simulink subsystem "External_Forces"  (R2024a)
settings: Solver=VariableStepAuto  StartTime=0.0  StopTime=10.0  RelTol=1e-3
undefined symbols (not defined in the file): EXT, P0, P1, P10, P2, P3, P4, P5, P6, P7, P8, P9, Sim_param
settings Model: Creator=esben  LastModifiedBy=BP21JL
settings SolverCC: AlgebraicLoopSolver=TrustRegion
settings DebuggingCC: UnconnectedInputMsg=warning  UnconnectedOutputMsg=warning  UnconnectedLineMsg=warning
settings ModelReferenceCC: EnableRefExpFcnMdlSchedulingChecks=on
settings RTWCC: GPUComputeCapability=3.5  DLArmComputeVersion=19.05

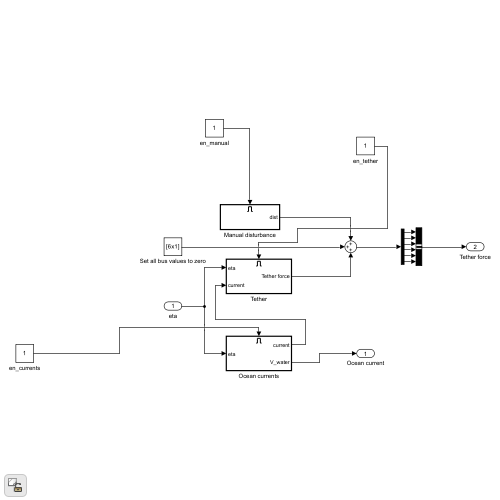
[thumbnail: Simulink's stored preview of the top-level diagram]
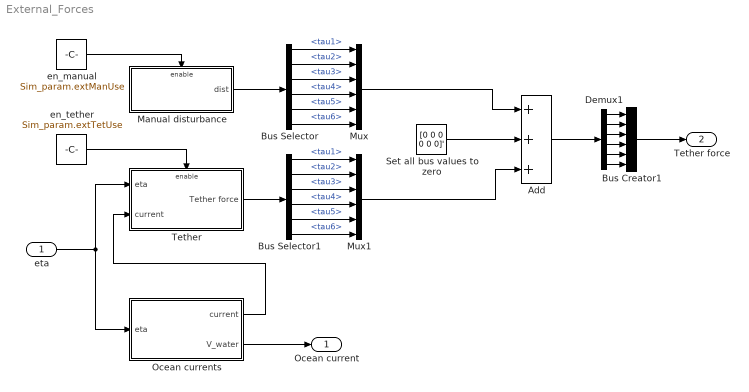
== system External_Forces ==
  eta : Inport
  Add : Sum  Inputs=+++
  Bus Creator1 : BusCreator  Inputs=6  OutDataTypeStr=Bus: tau
  Bus Selector : BusSelector  OutputSignals=tau1,tau2,tau3,tau4,tau5,tau6
  Bus Selector1 : BusSelector  OutputSignals=tau1,tau2,tau3,tau4,tau5,tau6
  Demux1 : Demux  Outputs=6
  Manual disturbance : Subsystem  TreatAsAtomicUnit=on
  Mux : Mux  Inputs=6
  Mux1 : Mux  Inputs=6
  Ocean currents : Subsystem  TreatAsAtomicUnit=on
  Set all bus values to zero : Constant  Value=[0 0 0 0 0 0]'
  Tether : Subsystem  TreatAsAtomicUnit=on
  en_manual : Constant  Value=Sim_param.extManUse
  en_tether : Constant  Value=Sim_param.extTetUse
  Ocean current : Outport
  Tether force : Outport  Port=2
  wires:
  eta/1 -> Tether/1(eta), Ocean currents/1(eta)
  Manual disturbance/1(dist) -> Bus Selector/1
  Demux1/4 -> Bus Creator1/4
  Demux1/2 -> Bus Creator1/2
  Demux1/5 -> Bus Creator1/5
  Demux1/1 -> Bus Creator1/1
  Bus Creator1/1 -> Tether force/1
  Demux1/6 -> Bus Creator1/6
  Demux1/3 -> Bus Creator1/3
  Ocean currents/1(current) -> Tether/2(current)
  Ocean currents/2(V_water) -> Ocean current/1
  en_tether/1 -> Tether/Enable
  en_manual/1 -> Manual disturbance/Enable
  Tether/1(Tether force) -> Bus Selector1/1
  Bus Selector1/1 -> Mux1/1  "<tau1>"
  Bus Selector1/2 -> Mux1/2  "<tau2>"
  Bus Selector1/3 -> Mux1/3  "<tau3>"
  Bus Selector1/4 -> Mux1/4  "<tau4>"
  Bus Selector1/5 -> Mux1/5  "<tau5>"
  Bus Selector1/6 -> Mux1/6  "<tau6>"
  Bus Selector/1 -> Mux/1  "<tau1>"
  Bus Selector/2 -> Mux/2  "<tau2>"
  Bus Selector/3 -> Mux/3  "<tau3>"
  Bus Selector/4 -> Mux/4  "<tau4>"
  Bus Selector/5 -> Mux/5  "<tau5>"
  Bus Selector/6 -> Mux/6  "<tau6>"
  Set all bus values to zero/1 -> Add/2
  Mux/1 -> Add/1
  Mux1/1 -> Add/3
  Add/1 -> Demux1/1

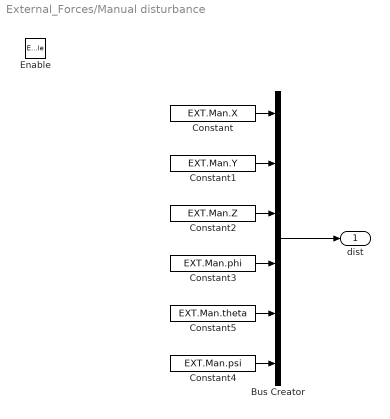
== system External_Forces/Manual disturbance ==
  Enable : EnablePort
  Bus Creator : BusCreator  Inputs=6  OutDataTypeStr=Bus: tau
      settings: InheritFromInputs=off
  Constant : Constant  Value=EXT.Man.X
  Constant1 : Constant  Value=EXT.Man.Y
  Constant2 : Constant  Value=EXT.Man.Z
  Constant3 : Constant  Value=EXT.Man.phi
  Constant4 : Constant  Value=EXT.Man.psi
  Constant5 : Constant  Value=EXT.Man.theta
  dist : Outport  OutDataTypeStr=Bus: tau
  wires:
  Constant1/1 -> Bus Creator/2
  Constant2/1 -> Bus Creator/3
  Constant5/1 -> Bus Creator/5
  Constant/1 -> Bus Creator/1
  Constant4/1 -> Bus Creator/6
  Constant3/1 -> Bus Creator/4
  Bus Creator/1 -> dist/1

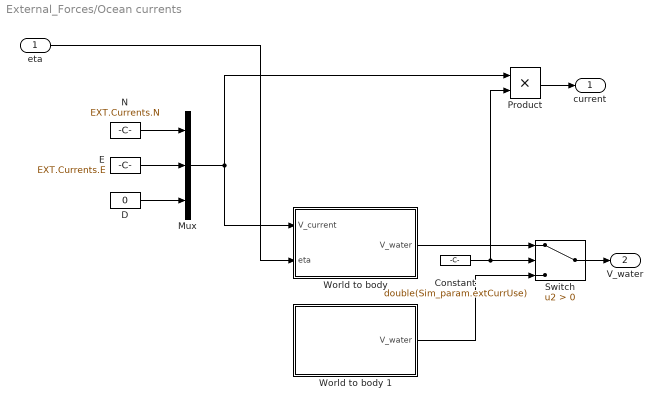
== system External_Forces/Ocean currents ==
  eta : Inport
  Constant : Constant  Value=double(Sim_param.extCurrUse)
  D : Constant  Value=0
  E : Constant  Value=EXT.Currents.E
  Mux : Mux  Inputs=3
  N : Constant  Value=EXT.Currents.N
  Product : Product
  Switch : Switch  Criteria=u2 > Threshold  SaturateOnIntegerOverflow=off  InputSameDT=off
  "World to body " : MATLAB Function  TreatAsAtomicUnit=on
  World to body 1 : MATLAB Function  TreatAsAtomicUnit=on
  current : Outport
  V_water : Outport  Port=2
  wires:
  Switch/1 -> V_water/1
  N/1 -> Mux/1
  eta/1 -> "World to body "/2(eta)
  World to body 1/1(V_water) -> Switch/3
  E/1 -> Mux/2
  "World to body "/1(V_water) -> Switch/1
  Constant/1 -> Switch/2, Product/2
  Product/1 -> current/1
  Mux/1 -> "World to body "/1(V_current), Product/1
  D/1 -> Mux/3

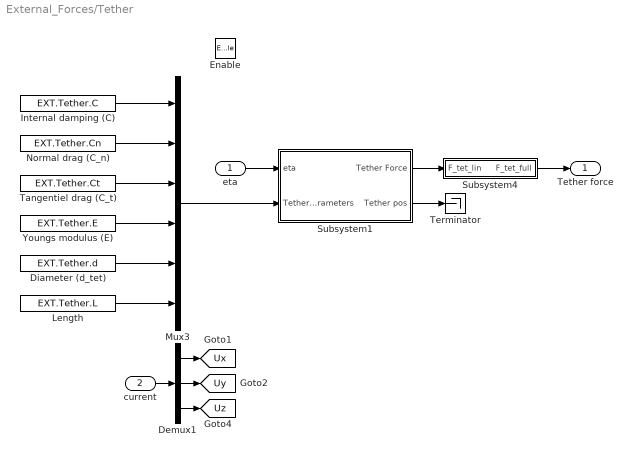
== system External_Forces/Tether ==
  eta : Inport
  current : Inport  Port=2
  Enable : EnablePort
  Demux1 : Demux  Outputs=3
  Diameter (d_tet) : Constant  Value=EXT.Tether.d
  Internal damping (C) : Constant  Value=EXT.Tether.C
  Length : Constant  Value=EXT.Tether.L
  Mux3 : Mux  Inputs=6
  Normal drag (C_n) : Constant  Value=EXT.Tether.Cn
  Subsystem1 : Subsystem
  Subsystem4 : Subsystem
  Tangentiel drag (C_t) : Constant  Value=EXT.Tether.Ct
  Terminator : Terminator
  Youngs modulus (E) : Constant  Value=EXT.Tether.E
  Tether force : Outport  OutDataTypeStr=Bus: tau
  tag scope: Ux=global, Uy=global, Uz=global
  wires:
  Diameter (d_tet)/1 -> Mux3/5
  Length/1 -> Mux3/6
  Demux1/3 -> [Uz]
  Internal damping (C)/1 -> Mux3/1
  Demux1/2 -> [Uy]
  current/1 -> Demux1/1
  Subsystem4/1(F_tet_full) -> Tether force/1
  Subsystem1/2(Tether pos) -> Terminator/1
  Normal drag (C_n)/1 -> Mux3/2
  eta/1 -> Subsystem1/1(eta)
  Mux3/1 -> Subsystem1/2(Tether_Parameters)
  Tangentiel drag (C_t)/1 -> Mux3/3
  Subsystem1/1(Tether Force) -> Subsystem4/1(F_tet_lin)
  Youngs modulus (E)/1 -> Mux3/4
  Demux1/1 -> [Ux]

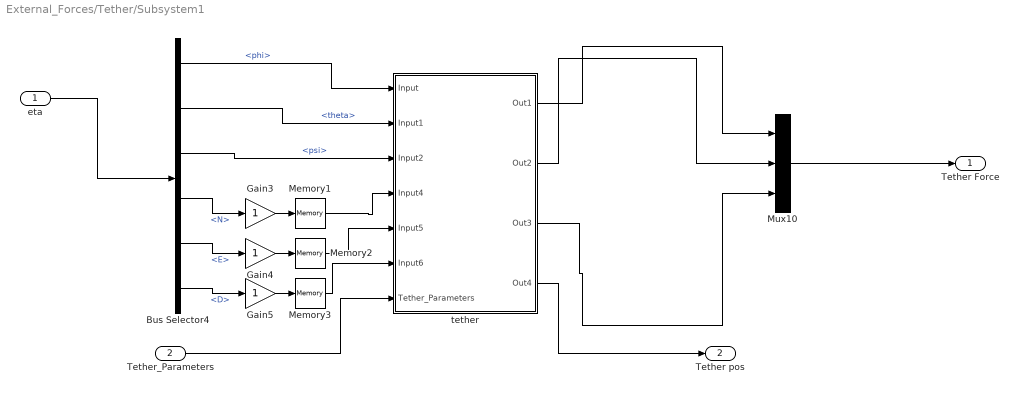
== system External_Forces/Tether/Subsystem1 ==
  eta : Inport
  Tether_Parameters : Inport  Port=2
  Bus Selector4 : BusSelector  OutputSignals=phi,theta,psi,N,E,D
  Gain3 : Gain
  Gain4 : Gain
  Gain5 : Gain
  Memory1 : Memory  InitialCondition=P10(1)
  Memory2 : Memory  InitialCondition=P10(2)
  Memory3 : Memory  InitialCondition=P10(3)
  Mux10 : Mux  Inputs=3
  tether : Subsystem
  Tether Force : Outport
  Tether pos : Outport  Port=2
  wires:
  eta/1 -> Bus Selector4/1
  Bus Selector4/6 -> Gain5/1  "<D>"
  Bus Selector4/5 -> Gain4/1  "<E>"
  Bus Selector4/4 -> Gain3/1  "<N>"
  tether/4(Out4) -> Tether pos/1
  Mux10/1 -> Tether Force/1
  tether/3(Out3) -> Mux10/3
  tether/2(Out2) -> Mux10/2
  tether/1(Out1) -> Mux10/1
  Gain5/1 -> Memory3/1
  Gain4/1 -> Memory2/1
  Gain3/1 -> Memory1/1
  Tether_Parameters/1 -> tether/7(Tether_Parameters)
  Bus Selector4/3 -> tether/3(Input2)  "<psi>"
  Bus Selector4/2 -> tether/2(Input1)  "<theta>"
  Bus Selector4/1 -> tether/1(Input)  "<phi>"
  Memory1/1 -> tether/4(Input4)
  Memory2/1 -> tether/5(Input5)
  Memory3/1 -> tether/6(Input6)

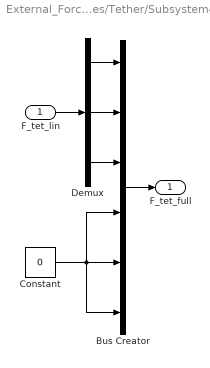
== system External_Forces/Tether/Subsystem4 ==
  F_tet_lin : Inport
  Bus Creator : BusCreator  Inputs=6  OutDataTypeStr=Bus: tau
      settings: InheritFromInputs=off
  Constant : Constant  Value=0
  Demux : Demux  Outputs=3
  F_tet_full : Outport  OutDataTypeStr=Bus: tau
  wires:
  F_tet_lin/1 -> Demux/1
  Demux/3 -> Bus Creator/3
  Demux/2 -> Bus Creator/2
  Demux/1 -> Bus Creator/1
  Bus Creator/1 -> F_tet_full/1
  Constant/1 -> Bus Creator/5, Bus Creator/4, Bus Creator/6

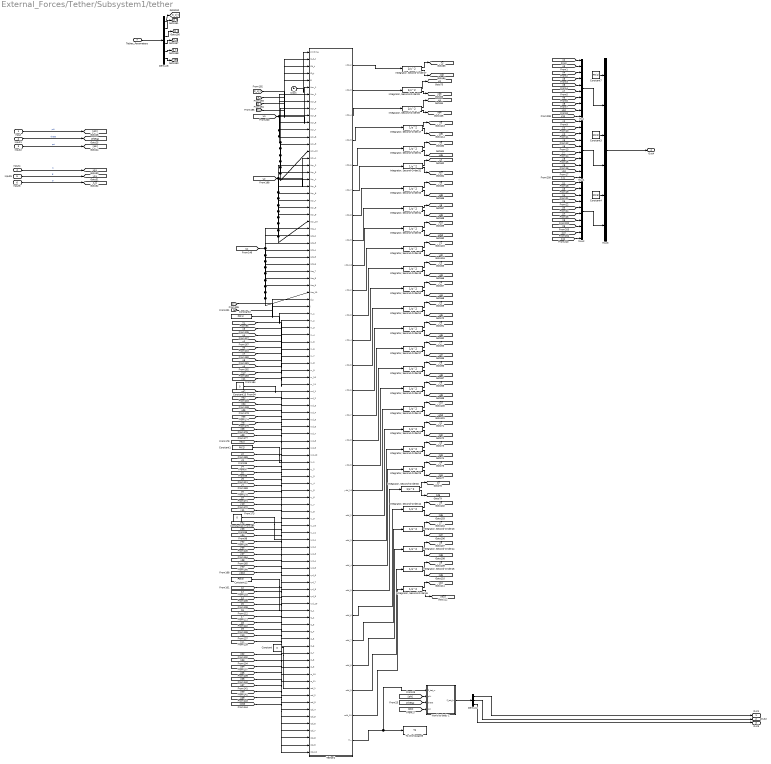
== system External_Forces/Tether/Subsystem1/tether ==
  Input : Inport
  Input1 : Inport  Port=2
  Input2 : Inport  Port=3
  Input4 : Inport  Port=4
  Input5 : Inport  Port=5
  Input6 : Inport  Port=6
  Tether_Parameters : Inport  Port=7
  Clock : Clock
  Constant : Constant  Value=0
  Constant1 : Constant  Value=P0(2)
  Constant10 : Constant  Value=0
  Constant12 : Constant  Value=P0(3)
  Constant13 : Constant  Value=0
  Constant2 : Constant  Value=P0(1)
  Constant3 : Constant  Value=P0(2)
  Constant4 : Constant  Value=P0(3)
  Constant7 : Constant  Value=P0(1)
  Demux4 : Demux  Outputs=3
  Demux6 : Demux  Outputs=6
  "Integrator, Second-Order27" : SecondOrderIntegrator  ICX=P1(1)
  "Integrator, Second-Order28" : SecondOrderIntegrator  ICX=P2(1)
  "Integrator, Second-Order29" : SecondOrderIntegrator  ICX=P3(3)
  "Integrator, Second-Order30" : SecondOrderIntegrator  ICX=P4(3)
  "Integrator, Second-Order31" : SecondOrderIntegrator  ICX=P5(1)
  "Integrator, Second-Order32" : SecondOrderIntegrator  ICX=P6(1)
  "Integrator, Second-Order33" : SecondOrderIntegrator  ICX=P7(1)
  "Integrator, Second-Order34" : SecondOrderIntegrator  ICX=P8(1)  UpperLimitX=100  LowerLimitX=-100  UpperLimitDXDT=10  LowerLimitDXDT=-10
  "Integrator, Second-Order35" : SecondOrderIntegrator  ICX=P9(1)
  "Integrator, Second-Order36" : SecondOrderIntegrator  ICX=P5(2)
  "Integrator, Second-Order37" : SecondOrderIntegrator  ICX=P6(2)
  "Integrator, Second-Order38" : SecondOrderIntegrator  ICX=P7(2)
  "Integrator, Second-Order39" : SecondOrderIntegrator  ICX=P3(1)
  "Integrator, Second-Order40" : SecondOrderIntegrator  ICX=P8(2)
  "Integrator, Second-Order41" : SecondOrderIntegrator  ICX=P9(2)
  "Integrator, Second-Order42" : SecondOrderIntegrator  ICX=P5(3)
  "Integrator, Second-Order43" : SecondOrderIntegrator  ICX=P6(3)
  "Integrator, Second-Order44" : SecondOrderIntegrator  ICX=P7(3)
  "Integrator, Second-Order45" : SecondOrderIntegrator  ICX=P8(3)
  "Integrator, Second-Order46" : SecondOrderIntegrator  ICX=P9(3)
  "Integrator, Second-Order47" : SecondOrderIntegrator  ICX=P4(1)
  "Integrator, Second-Order48" : SecondOrderIntegrator  ICX=P1(2)
  "Integrator, Second-Order49" : SecondOrderIntegrator  ICX=P2(2)
  "Integrator, Second-Order50" : SecondOrderIntegrator  ICX=P3(2)
  "Integrator, Second-Order51" : SecondOrderIntegrator  ICX=P4(2)
  "Integrator, Second-Order52" : SecondOrderIntegrator  ICX=P1(3)
  "Integrator, Second-Order53" : SecondOrderIntegrator  ICX=P2(3)
  Mux : Mux  Inputs=10
  Mux1 : Mux  Inputs=10
  Mux2 : Mux  Inputs=10
  Mux3 : Mux  Inputs=6
  Tether2 : MATLAB Function  TreatAsAtomicUnit=on
  To Workspace3 : ToWorkspace  VariableName=T2  SaveFormat=Timeseries  SampleTime=-1
  World to body 1 : MATLAB Function  TreatAsAtomicUnit=on
  Out1 : Outport
  Out2 : Outport  Port=2
  Out3 : Outport  Port=3
  Out4 : Outport  Port=4
  tag scope: C_d_t=global, Cd_t=global, Ct_t=global, Em_t=global, I_tet=global, d_t=global, x10=global, x11=global, x2=global, x3=global, x4=global, x5=global, x6=global, x7=global, x8=global, x9=global, xd10=global, xd2=global, xd3=global, xd4=global, xd5=global, xd6=global, xd7=global, xd8=global, xd9=global, y10=global, y11=global, y2=global, y3=global, y4=global, y5=global, y6=global, y7=global, y8=global, y9=global, yd10=global, yd2=global, yd3=global, yd4=global, yd5=global, yd6=global, yd7=global, yd8=global, yd9=global, z10=global, z11=global, z2=global, z3=global, z4=global, z5=global, z6=global, z7=global, z8=global, z9=global, zd10=global, zd2=global, zd3=global, zd4=global, zd5=global, zd6=global, zd7=global, zd8=global, zd9=global
  wires:
  Clock/1 -> Tether2/1(simtime)
  Constant4/1 -> Mux3/5
  Constant3/1 -> Mux3/3
  Constant7/1 -> Mux3/1
  Mux3/1 -> Out4/1
  Mux2/1 -> Mux3/6
  Mux1/1 -> Mux3/4
  Mux/1 -> Mux3/2
  [z11] -> Mux2/10
  [y11] -> Mux1/10
  [x11] -> Mux/10
  [z2] -> Mux2/1
  [z6] -> Mux2/5
  [z10] -> Mux2/9
  [z7] -> Mux2/6
  [z8] -> Mux2/7
  [z3] -> Mux2/2
  [z4] -> Mux2/3
  [z5] -> Mux2/4
  [z9] -> Mux2/8
  [y2] -> Mux1/1
  [y6] -> Mux1/5
  [y10] -> Mux1/9
  [y7] -> Mux1/6
  [y8] -> Mux1/7
  [y3] -> Mux1/2
  [y4] -> Mux1/3
  [y5] -> Mux1/4
  [y9] -> Mux1/8
  [x10] -> Mux/9
  [x9] -> Mux/8
  [x8] -> Mux/7
  [x7] -> Mux/6
  [x6] -> Mux/5
  [x5] -> Mux/4
  [x4] -> Mux/3
  [x3] -> Mux/2
  [x2] -> Mux/1
  Constant13/1 -> Tether2/49(rxd_1)
  Constant10/1 -> Tether2/70(ryd_1)
  Constant/1 -> Tether2/91(rzd_1)
  Tether2/4(xdd_5) -> "Integrator, Second-Order47"/1
  Tether2/3(xdd_4) -> "Integrator, Second-Order39"/1
  Tether2/2(xdd_3) -> "Integrator, Second-Order28"/1
  Tether2/1(xdd_2) -> "Integrator, Second-Order27"/1
  Tether2/27(zdd_10) -> "Integrator, Second-Order46"/1
  Tether2/26(zdd_9) -> "Integrator, Second-Order45"/1
  Tether2/25(zdd_8) -> "Integrator, Second-Order44"/1
  Tether2/24(zdd_7) -> "Integrator, Second-Order43"/1
  Tether2/23(zdd_6) -> "Integrator, Second-Order42"/1
  Tether2/22(zdd_5) -> "Integrator, Second-Order30"/1
  Tether2/21(zdd_4) -> "Integrator, Second-Order29"/1
  Tether2/20(zdd_3) -> "Integrator, Second-Order53"/1
  Tether2/19(zdd_2) -> "Integrator, Second-Order52"/1
  Tether2/18(ydd_10) -> "Integrator, Second-Order41"/1
  Tether2/17(ydd_9) -> "Integrator, Second-Order40"/1
  Tether2/16(ydd_8) -> "Integrator, Second-Order38"/1
  Tether2/15(ydd_7) -> "Integrator, Second-Order37"/1
  Tether2/14(ydd_6) -> "Integrator, Second-Order36"/1
  Tether2/13(ydd_5) -> "Integrator, Second-Order51"/1
  Tether2/12(ydd_4) -> "Integrator, Second-Order50"/1
  Tether2/11(ydd_3) -> "Integrator, Second-Order49"/1
  Tether2/10(ydd_2) -> "Integrator, Second-Order48"/1
  Tether2/9(xdd_10) -> "Integrator, Second-Order35"/1
  Tether2/8(xdd_9) -> "Integrator, Second-Order34"/1
  Tether2/7(xdd_8) -> "Integrator, Second-Order33"/1
  Tether2/6(xdd_7) -> "Integrator, Second-Order32"/1
  Tether2/5(xdd_6) -> "Integrator, Second-Order31"/1
  Demux6/1 -> [C_d_t]
  [C_d_t] -> Tether2/2(C_d_t)
  Demux6/4 -> [Em_t]
  Demux6/5 -> [d_t]
  Demux6/2 -> [Cd_t]
  Tether_Parameters/1 -> Demux6/1
  Demux6/3 -> [Ct_t]
  Demux6/6 -> [I_tet]
  [Em_t] -> Tether2/5(E)
  [Ct_t] -> Tether2/4(Ct_t)
  [Cd_t] -> Tether2/3(Cd_t)
  [d_t] -> Tether2/36(d_t)
  [Uy] -> Tether2/16(Ucy_1), Tether2/17(Ucy_2), Tether2/18(Ucy_3), Tether2/19(Ucy_4), Tether2/20(Ucy_5), Tether2/21(Ucy_6), Tether2/22(Ucy_7), Tether2/23(Ucy_8), Tether2/24(Ucy_9), Tether2/25(Ucy_10)
  Demux4/2 -> Out2/1
  Demux4/3 -> Out3/1
  Demux4/1 -> Out1/1
  Tether2/28(Tix) -> To Workspace3/1, World to body 1/1(F_tet_w)
  [phi] -> World to body 1/2(phi)
  [theta] -> World to body 1/3(theta)
  World to body 1/1(F_tet_b) -> Demux4/1
  [psi] -> World to body 1/4(psi)
  [I_tet] -> Tether2/37(l)
  [Ux] -> Tether2/6(Ucx_1), Tether2/7(Ucx_2), Tether2/8(Ucx_3), Tether2/9(Ucx_4), Tether2/10(Ucx_5), Tether2/11(Ucx_6), Tether2/12(Ucx_7), Tether2/13(Ucx_8), Tether2/14(Ucx_9), Tether2/15(Ucx_10)
  [x9] -> Tether2/46(rx_9)
  "Integrator, Second-Order42"/1 -> [z6]
  [y3] -> Tether2/61(ry_3)
  "Integrator, Second-Order53"/2 -> [zd3]
  "Integrator, Second-Order43"/2 -> [zd7]
  [xd2] -> Tether2/50(rxd_2)
  "Integrator, Second-Order38"/2 -> [yd8]
  "Integrator, Second-Order39"/2 -> [xd4]
  "Integrator, Second-Order33"/1 -> [x8]
  [x11] -> Tether2/48(rx_11)
  [Uz] -> Tether2/26(Ucz_1), Tether2/27(Ucz_2), Tether2/28(Ucz_3), Tether2/29(Ucz_4), Tether2/30(Ucz_5), Tether2/31(Ucz_6), Tether2/32(Ucz_7), Tether2/33(Ucz_8), Tether2/34(Ucz_9), Tether2/35(Ucz_10)
  [x2] -> Tether2/39(rx_2)
  [x10] -> Tether2/47(rx_10)
  "Integrator, Second-Order42"/2 -> [zd6]
  [z10] -> Tether2/89(rz_10)
  [y8] -> Tether2/66(ry_8)
  [yd9] -> Tether2/78(ryd_9)
  [xd7] -> Tether2/55(rxd_7)
  [y11] -> Tether2/69(ry_11)
  "Integrator, Second-Order27"/2 -> [xd2]
  "Integrator, Second-Order49"/2 -> [yd3]
  [y2] -> Tether2/60(ry_2)
  "Integrator, Second-Order30"/2 -> [zd5]
  [xd3] -> Tether2/51(rxd_3)
  "Integrator, Second-Order35"/1 -> [x10]
  [zd2] -> Tether2/92(rzd_2)
  [yd6] -> Tether2/75(ryd_6)
  [y7] -> Tether2/65(ry_7)
  [x5] -> Tether2/42(rx_5)
  [xd10] -> Tether2/58(rxd_10)
  [x8] -> Tether2/45(rx_8)
  [zd8] -> Tether2/98(rzd_8)
  [x6] -> Tether2/43(rx_6)
  [yd4] -> Tether2/73(ryd_4)
  "Integrator, Second-Order34"/2 -> [xd9]
  [xd6] -> Tether2/54(rxd_6)
  [z2] -> Tether2/81(rz_2)
  [z7] -> Tether2/86(rz_7)
  "Integrator, Second-Order39"/1 -> [x4]
  [z5] -> Tether2/84(rz_5)
  "Integrator, Second-Order28"/1 -> [x3]
  "Integrator, Second-Order44"/1 -> [z8]
  "Integrator, Second-Order34"/1 -> [x9]
  Constant2/1 -> Tether2/38(rx_1)
  "Integrator, Second-Order51"/1 -> [y5]
  "Integrator, Second-Order43"/1 -> [z7]
  "Integrator, Second-Order40"/2 -> [yd9]
  [z6] -> Tether2/85(rz_6)
  "Integrator, Second-Order37"/1 -> [y7]
  [xd8] -> Tether2/56(rxd_8)
  "Integrator, Second-Order45"/1 -> [z9]
  [x4] -> Tether2/41(rx_4)
  "Integrator, Second-Order32"/2 -> [xd7]
  "Integrator, Second-Order49"/1 -> [y3]
  "Integrator, Second-Order47"/1 -> [x5]
  "Integrator, Second-Order36"/2 -> [yd6]
  "Integrator, Second-Order51"/2 -> [yd5]
  [yd2] -> Tether2/71(ryd_2)
  "Integrator, Second-Order48"/2 -> [yd2]
  "Integrator, Second-Order27"/1 -> [x2]
  "Integrator, Second-Order40"/1 -> [y9]
  "Integrator, Second-Order44"/2 -> [zd8]
  [yd5] -> Tether2/74(ryd_5)
  [x3] -> Tether2/40(rx_3)
  [zd9] -> Tether2/99(rzd_9)
  [x7] -> Tether2/44(rx_7)
  "Integrator, Second-Order37"/2 -> [yd7]
  [xd4] -> Tether2/52(rxd_4)
  [z3] -> Tether2/82(rz_3)
  "Integrator, Second-Order31"/1 -> [x6]
  [y4] -> Tether2/62(ry_4)
  "Integrator, Second-Order47"/2 -> [xd5]
  [z11] -> Tether2/90(rz_11)
  [zd4] -> Tether2/94(rzd_4)
  "Integrator, Second-Order45"/2 -> [zd9]
  "Integrator, Second-Order48"/1 -> [y2]
  [y10] -> Tether2/68(ry_10)
  [z4] -> Tether2/83(rz_4)
  [yd10] -> Tether2/79(ryd_10)
  "Integrator, Second-Order46"/2 -> [zd10]
  [y9] -> Tether2/67(ry_9)
  Constant1/1 -> Tether2/59(ry_1)
  "Integrator, Second-Order30"/1 -> [z5]
  "Integrator, Second-Order41"/1 -> [y10]
  [yd8] -> Tether2/77(ryd_8)
  "Integrator, Second-Order33"/2 -> [xd8]
  "Integrator, Second-Order31"/2 -> [xd6]
  "Integrator, Second-Order38"/1 -> [y8]
  [z9] -> Tether2/88(rz_9)
  "Integrator, Second-Order41"/2 -> [yd10]
  [yd3] -> Tether2/72(ryd_3)
  [zd6] -> Tether2/96(rzd_6)
  [xd9] -> Tether2/57(rxd_9)
  [zd10] -> Tether2/100(rzd_10)
  [zd5] -> Tether2/95(rzd_5)
  "Integrator, Second-Order53"/1 -> [z3]
  "Integrator, Second-Order50"/2 -> [yd4]
  [xd5] -> Tether2/53(rxd_5)
  [y6] -> Tether2/64(ry_6)
  "Integrator, Second-Order50"/1 -> [y4]
  [z8] -> Tether2/87(rz_8)
  "Integrator, Second-Order52"/2 -> [zd2]
  [y5] -> Tether2/63(ry_5)
  "Integrator, Second-Order35"/2 -> [xd10]
  "Integrator, Second-Order29"/1 -> [z4]
  "Integrator, Second-Order29"/2 -> [zd4]
  Constant12/1 -> Tether2/80(rz_1)
  [zd3] -> Tether2/93(rzd_3)
  [yd7] -> Tether2/76(ryd_7)
  "Integrator, Second-Order32"/1 -> [x7]
  "Integrator, Second-Order36"/1 -> [y6]
  "Integrator, Second-Order28"/2 -> [xd3]
  [zd7] -> Tether2/97(rzd_7)
  "Integrator, Second-Order52"/1 -> [z2]
  "Integrator, Second-Order46"/1 -> [z10]
  Input6/1 -> [z11]  "D"
  Input5/1 -> [y11]  "E"
  Input4/1 -> [x11]  "N"
  Input2/1 -> [psi]  "psi"
  Input1/1 -> [theta]  "theta"
  Input/1 -> [phi]  "phi"

== matlab function External_Forces/Tether/Subsystem1/tether/Tether2 ==
  data: simtime input; C_d_t input; xdd_2 output; Cd_t input; Ct_t input; E input; Ucx_1 input; Ucx_2 input; Ucx_3 input; Ucx_4 input; Ucx_5 input; Ucx_6 input; Ucx_7 input; Ucx_8 input; Ucx_9 input; Ucx_10 input; Ucy_1 input; Ucy_2 input; Ucy_3 input; Ucy_4 input; Ucy_5 input; Ucy_6 input; Ucy_7 input; Ucy_8 input; Ucy_9 input; Ucy_10 input; Ucz_1 input; Ucz_2 input; Ucz_3 input; Ucz_4 input; Ucz_5 input; Ucz_6 input; Ucz_7 input; Ucz_8 input; Ucz_9 input; Ucz_10 input; d_t input; l input; rx_1 input; rx_2 input; rx_3 input; rx_4 input; rx_5 input; rx_6 input; rx_7 input; rx_8 input; rx_9 input; rx_10 input; rx_11 input; rxd_1 input; rxd_2 input; rxd_3 input; rxd_4 input; rxd_5 input; rxd_6 input; rxd_7 input; rxd_8 input; rxd_9 input; rxd_10 input; ry_1 input; ry_2 input; ry_3 input; ry_4 input; ry_5 input; ry_6 input; ry_7 input; ry_8 input; ry_9 input; ry_10 input; ry_11 input; ryd_1 input; ryd_2 input; ryd_3 input; ryd_4 input; ryd_5 input; ryd_6 input; ryd_7 input; ryd_8 input; ryd_9 input; ryd_10 input; rz_1 input; rz_2 input; rz_3 input; rz_4 input; rz_5 input; rz_6 input; rz_7 input; rz_8 input; rz_9 input; rz_10 input; rz_11 input; rzd_1 input; rzd_2 input; rzd_3 input; rzd_4 input; rzd_5 input; rzd_6 input; rzd_7 input; rzd_8 input; rzd_9 input; rzd_10 input; xdd_3 output; xdd_4 output; xdd_5 output; xdd_6 output; xdd_7 output; xdd_8 output; xdd_9 output; xdd_10 output; ydd_2 output; ydd_3 output; ydd_4 output; ydd_5 output; ydd_6 output; ydd_7 output; ydd_8 output; ydd_9 output; ydd_10 output; zdd_2 output; zdd_3 output; zdd_4 output; zdd_5 output; zdd_6 output; zdd_7 output; zdd_8 output; zdd_9 output; zdd_10 output; Tix output
function [xdd_2,xdd_3,xdd_4,xdd_5,xdd_6,xdd_7,xdd_8,xdd_9,xdd_10,ydd_2,ydd_3,ydd_4,ydd_5,ydd_6,ydd_7,ydd_8,ydd_9,ydd_10,zdd_2,zdd_3,zdd_4,zdd_5,zdd_6,zdd_7,zdd_8,zdd_9,zdd_10,Tix] = Tether(simtime,C_d_t,Cd_t,Ct_t,E,Ucx_1,Ucx_2,Ucx_3,Ucx_4,Ucx_5,Ucx_6,Ucx_7,Ucx_8,Ucx_9,Ucx_10,Ucy_1,Ucy_2,Ucy_3,Ucy_4,Ucy_5,Ucy_6,Ucy_7,Ucy_8,Ucy_9,Ucy_10,Ucz_1,Ucz_2,Ucz_3,Ucz_4,Ucz_5,Ucz_6,Ucz_7,Ucz_8,Ucz_9,Ucz_10,d_t,l,rx_1,rx_2,rx_3,rx_4,rx_5,rx_6,rx_7,rx_8,rx_9,rx_10,rx_11,rxd_1,rxd_2,rxd_3,rxd_4,rxd_5,rxd_6,rxd_7,rxd_8,rxd_9,rxd_10,ry_1,ry_2,ry_3,ry_4,ry_5,ry_6,ry_7,ry_8,ry_9,ry_10,ry_11,ryd_1,ryd_2,ryd_3,ryd_4,ryd_5,ryd_6,ryd_7,ryd_8,ryd_9,ryd_10,rz_1,rz_2,rz_3,rz_4,rz_5,rz_6,rz_7,rz_8,rz_9,rz_10,rz_11,rzd_1,rzd_2,rzd_3,rzd_4,rzd_5,rzd_6,rzd_7,rzd_8,rzd_9,rzd_10)
%#codegen

%    This function was generated by the Symbolic Math Toolbox version 8.6.
%    17-Mar-2022 13:31:39
%if simtime > 0.5

t2 = d_t.^2;
t3 = -Ucx_2;
t4 = -Ucx_3;
t5 = -Ucx_4;
t6 = -Ucx_5;
t7 = -Ucx_6;
t8 = -Ucx_7;
t9 = -Ucx_8;
t10 = -Ucx_9;
t11 = -Ucx_10;
t12 = -Ucy_2;
t13 = -Ucy_3;
t14 = -Ucy_4;
t15 = -Ucy_5;
t16 = -Ucy_6;
t17 = -Ucy_7;
t18 = -Ucy_8;
t19 = -Ucy_9;
t20 = -Ucy_10;
t21 = -Ucz_2;
t22 = -Ucz_3;
t23 = -Ucz_4;
t24 = -Ucz_5;
t25 = -Ucz_6;
t26 = -Ucz_7;
t27 = -Ucz_8;
t28 = -Ucz_9;
t29 = -Ucz_10;
t30 = 1.0./l;
t31 = -rx_2;
t32 = -rx_3;
t33 = -rx_4;
t34 = -rx_5;
t35 = -rx_6;
t36 = -rx_7;
t37 = -rx_8;
t38 = -rx_9;
t39 = -rx_10;
t40 = -rx_11;
t41 = -rxd_2;
t42 = -rxd_3;
t43 = -rxd_4;
t44 = -rxd_5;
t45 = -rxd_6;
t46 = -rxd_7;
t47 = -rxd_8;
t48 = -rxd_9;
t49 = -rxd_10;
t50 = -ry_2;
t51 = -ry_3;
t52 = -ry_4;
t53 = -ry_5;
t54 = -ry_6;
t55 = -ry_7;
t56 = -ry_8;
t57 = -ry_9;
t58 = -ry_10;
t59 = -ry_11;
t60 = -ryd_2;
t61 = -ryd_3;
t62 = -ryd_4;
t63 = -ryd_5;
t64 = -ryd_6;
t65 = -ryd_7;
t66 = -ryd_8;
t67 = -ryd_9;
t68 = -ryd_10;
t69 = -rz_2;
t70 = -rz_3;
t71 = -rz_4;
t72 = -rz_5;
t73 = -rz_6;
t74 = -rz_7;
t75 = -rz_8;
t76 = -rz_9;
t77 = -rz_10;
t78 = -rz_11;
t79 = -rzd_2;
t80 = -rzd_3;
t81 = -rzd_4;
t82 = -rzd_5;
t83 = -rzd_6;
t84 = -rzd_7;
t85 = -rzd_8;
t86 = -rzd_9;
t87 = -rzd_10;
t260 = l.*4.3e-3;
t88 = Ucx_2+t41;
t89 = Ucx_3+t42;
t90 = Ucx_4+t43;
t91 = Ucx_5+t44;
t92 = Ucx_6+t45;
t93 = Ucx_7+t46;
t94 = Ucx_8+t47;
t95 = Ucx_9+t48;
t96 = Ucx_10+t49;
t97 = Ucy_2+t60;
t98 = Ucy_3+t61;
t99 = Ucy_4+t62;
t100 = Ucy_5+t63;
t101 = Ucy_6+t64;
t102 = Ucy_7+t65;
t103 = Ucy_8+t66;
t104 = Ucy_9+t67;
t105 = Ucy_10+t68;
t106 = Ucz_2+t79;
t107 = Ucz_3+t80;
t108 = Ucz_4+t81;
t109 = Ucz_5+t82;
t110 = Ucz_6+t83;
t111 = Ucz_7+t84;
t112 = Ucz_8+t85;
t113 = Ucz_9+t86;
t114 = Ucz_10+t87;
t115 = rx_1+t31;
t116 = rx_2+t32;
t117 = rx_3+t33;
t118 = rx_4+t34;
t119 = rx_5+t35;
t120 = rx_6+t36;
t121 = rx_7+t37;
t122 = rx_8+t38;
t123 = rx_9+t39;
t124 = rx_10+t40;
t125 = rxd_1+t41;
t126 = rxd_2+t42;
t127 = rxd_3+t43;
t128 = rxd_4+t44;
t129 = rxd_5+t45;
t130 = rxd_6+t46;
t131 = rxd_7+t47;
t132 = rxd_8+t48;
t133 = rxd_9+t49;
t134 = ry_1+t50;
t135 = ry_2+t51;
t136 = ry_3+t52;
t137 = ry_4+t53;
t138 = ry_5+t54;
t139 = ry_6+t55;
t140 = ry_7+t56;
t141 = ry_8+t57;
t142 = ry_9+t58;
t143 = ry_10+t59;
t144 = ryd_1+t60;
t145 = ryd_2+t61;
t146 = ryd_3+t62;
t147 = ryd_4+t63;
t148 = ryd_5+t64;
t149 = ryd_6+t65;
t150 = ryd_7+t66;
t151 = ryd_8+t67;
t152 = ryd_9+t68;
t153 = rz_1+t69;
t154 = rz_2+t70;
t155 = rz_3+t71;
t156 = rz_4+t72;
t157 = rz_5+t73;
t158 = rz_6+t74;
t159 = rz_7+t75;
t160 = rz_8+t76;
t161 = rz_9+t77;
t162 = rz_10+t78;
t163 = rzd_1+t79;
t164 = rzd_2+t80;
t165 = rzd_3+t81;
t166 = rzd_4+t82;
t167 = rzd_5+t83;
t168 = rzd_6+t84;
t169 = rzd_7+t85;
t170 = rzd_8+t86;
t171 = rzd_9+t87;
t229 = l.*t2.*pi.*2.5e+1;
t172 = abs(t115);
t173 = abs(t116);
t174 = abs(t117);
t175 = abs(t118);
t176 = abs(t119);
t177 = abs(t120);
t178 = abs(t121);
t179 = abs(t122);
t180 = abs(t123);
t181 = abs(t124);
t182 = abs(t134);
t183 = abs(t135);
t184 = abs(t136);
t185 = abs(t137);
t186 = abs(t138);
t187 = abs(t139);
t188 = abs(t140);
t189 = abs(t141);
t190 = abs(t142);
t191 = abs(t143);
t192 = abs(t153);
t193 = abs(t154);
t194 = abs(t155);
t195 = abs(t156);
t196 = abs(t157);
t197 = abs(t158);
t198 = abs(t159);
t199 = abs(t160);
t200 = abs(t161);
t201 = abs(t162);
t202 = t115.^2;
t203 = t116.^2;
t204 = t117.^2;
t205 = t118.^2;
t206 = t119.^2;
t207 = t120.^2;
t208 = t121.^2;
t209 = t122.^2;
t210 = t123.^2;
t211 = t134.^2;
t212 = t135.^2;
t213 = t136.^2;
t214 = t137.^2;
t215 = t138.^2;
t216 = t139.^2;
t217 = t140.^2;
t218 = t141.^2;
t219 = t142.^2;
t220 = t153.^2;
t221 = t154.^2;
t222 = t155.^2;
t223 = t156.^2;
t224 = t157.^2;
t225 = t158.^2;
t226 = t159.^2;
t227 = t160.^2;
t228 = t161.^2;
t261 = rxd_1.*t30.*t115.*1.0e+1;
t262 = ryd_1.*t30.*t134.*1.0e+1;
t263 = rzd_1.*t30.*t153.*1.0e+1;
t264 = t229+t260;
t265 = t30.*t116.*t125.*1.0e+1;
t266 = t30.*t117.*t126.*1.0e+1;
t267 = t30.*t118.*t127.*1.0e+1;
t268 = t30.*t119.*t128.*1.0e+1;
t269 = t30.*t120.*t129.*1.0e+1;
t270 = t30.*t121.*t130.*1.0e+1;
t271 = t30.*t122.*t131.*1.0e+1;
t272 = t30.*t123.*t132.*1.0e+1;
t273 = t30.*t124.*t133.*1.0e+1;
t274 = t30.*t135.*t144.*1.0e+1;
t275 = t30.*t136.*t145.*1.0e+1;
t276 = t30.*t137.*t146.*1.0e+1;
t277 = t30.*t138.*t147.*1.0e+1;
t278 = t30.*t139.*t148.*1.0e+1;
t279 = t30.*t140.*t149.*1.0e+1;
t280 = t30.*t141.*t150.*1.0e+1;
t281 = t30.*t142.*t151.*1.0e+1;
t282 = t30.*t143.*t152.*1.0e+1;
t283 = t30.*t154.*t163.*1.0e+1;
t284 = t30.*t155.*t164.*1.0e+1;
t285 = t30.*t156.*t165.*1.0e+1;
t286 = t30.*t157.*t166.*1.0e+1;
t287 = t30.*t158.*t167.*1.0e+1;
t288 = t30.*t159.*t168.*1.0e+1;
t289 = t30.*t160.*t169.*1.0e+1;
t290 = t30.*t161.*t170.*1.0e+1;
t291 = t30.*t162.*t171.*1.0e+1;
t230 = t172.^2;
t231 = t173.^2;
t232 = t174.^2;
t233 = t175.^2;
t234 = t176.^2;
t235 = t177.^2;
t236 = t178.^2;
t237 = t179.^2;
t238 = t180.^2;
t239 = t181.^2;
t240 = t182.^2;
t241 = t183.^2;
t242 = t184.^2;
t243 = t185.^2;
t244 = t186.^2;
t245 = t187.^2;
t246 = t188.^2;
t247 = t189.^2;
t248 = t190.^2;
t249 = t191.^2;
t250 = t192.^2;
t251 = t193.^2;
t252 = t194.^2;
t253 = t195.^2;
t254 = t196.^2;
t255 = t197.^2;
t256 = t198.^2;
t257 = t199.^2;
t258 = t200.^2;
t259 = t201.^2;
t292 = 1.0./t264;
t363 = t261+t262+t263;
t415 = t265+t274+t283;
t416 = t266+t275+t284;
t417 = t267+t276+t285;
t418 = t268+t277+t286;
t419 = t269+t278+t287;
t420 = t270+t279+t288;
t421 = t271+t280+t289;
t422 = t272+t281+t290;
t423 = t273+t282+t291;
t293 = t230+t240+t250;
t294 = t231+t241+t251;
t295 = t232+t242+t252;
t296 = t233+t243+t253;
t297 = t234+t244+t254;
t298 = t235+t245+t255;
t299 = t236+t246+t256;
t300 = t237+t247+t257;
t301 = t238+t248+t258;
t302 = t239+t249+t259;
t303 = 1.0./t293;
t304 = 1.0./t294;
t306 = 1.0./t295;
t308 = 1.0./t296;
t310 = 1.0./t297;
t312 = 1.0./t298;
t314 = 1.0./t299;
t316 = 1.0./t300;
t318 = 1.0./t301;
t320 = 1.0./t302.^2;
t321 = sqrt(t294);
t322 = sqrt(t295);
t323 = sqrt(t296);
t324 = sqrt(t297);
t325 = sqrt(t298);
t326 = sqrt(t299);
t327 = sqrt(t300);
t328 = sqrt(t301);
t329 = sqrt(t302);
t330 = 1.0./sqrt(t293);
t305 = t304.^2;
t307 = t306.^2;
t309 = t308.^2;
t311 = t310.^2;
t313 = t312.^2;
t315 = t314.^2;
t317 = t316.^2;
t319 = t318.^2;
t331 = 1.0./t321;
t332 = 1.0./t322;
t333 = 1.0./t323;
t334 = 1.0./t324;
t335 = 1.0./t325;
t336 = 1.0./t326;
t337 = 1.0./t327;
t338 = 1.0./t328;
t339 = 1.0./t329;
t340 = (l.*t330)./1.0e+1;
t350 = Ucx_1.*t202.*t303;
t351 = Ucy_1.*t211.*t303;
t352 = Ucz_1.*t220.*t303;
t364 = t88.*t203.*t304;
t365 = t89.*t204.*t306;
t366 = t90.*t205.*t308;
t367 = t91.*t206.*t310;
t368 = t92.*t207.*t312;
t369 = t93.*t208.*t314;
t370 = t94.*t209.*t316;
t371 = t95.*t210.*t318;
t372 = t97.*t212.*t304;
t373 = t98.*t213.*t306;
t374 = t99.*t214.*t308;
t375 = t100.*t215.*t310;
t376 = t101.*t216.*t312;
t377 = t102.*t217.*t314;
t378 = t103.*t218.*t316;
t379 = t104.*t219.*t318;
t380 = t106.*t221.*t304;
t381 = t107.*t222.*t306;
t382 = t108.*t223.*t308;
t383 = t109.*t224.*t310;
t384 = t110.*t225.*t312;
t385 = t111.*t226.*t314;
t386 = t112.*t227.*t316;
t387 = t113.*t228.*t318;
t341 = (l.*t331)./1.0e+1;
t342 = (l.*t332)./1.0e+1;
t343 = (l.*t333)./1.0e+1;
t344 = (l.*t334)./1.0e+1;
t345 = (l.*t335)./1.0e+1;
t346 = (l.*t336)./1.0e+1;
t347 = (l.*t337)./1.0e+1;
t348 = (l.*t338)./1.0e+1;
t349 = (l.*t339)./1.0e+1;
t353 = t340-1.0;
t388 = rxd_2+t3+t350;
t389 = ryd_2+t12+t351;
t390 = rzd_2+t21+t352;
t391 = rxd_3+t4+t364;
t392 = rxd_4+t5+t365;
t393 = rxd_5+t6+t366;
t394 = rxd_6+t7+t367;
t395 = rxd_7+t8+t368;
t396 = rxd_8+t9+t369;
t397 = rxd_9+t10+t370;
t398 = rxd_10+t11+t371;
t399 = ryd_3+t13+t372;
t400 = ryd_4+t14+t373;
t401 = ryd_5+t15+t374;
t402 = ryd_6+t16+t375;
t403 = ryd_7+t17+t376;
t404 = ryd_8+t18+t377;
t405 = ryd_9+t19+t378;
t406 = ryd_10+t20+t379;
t407 = rzd_3+t22+t380;
t408 = rzd_4+t23+t381;
t409 = rzd_5+t24+t382;
t410 = rzd_6+t25+t383;
t411 = rzd_7+t26+t384;
t412 = rzd_8+t27+t385;
t413 = rzd_9+t28+t386;
t414 = rzd_10+t29+t387;
t451 = C_d_t.*t116.*t331.*t415;
t452 = C_d_t.*t117.*t332.*t416;
t453 = C_d_t.*t118.*t333.*t417;
t454 = C_d_t.*t119.*t334.*t418;
t455 = C_d_t.*t120.*t335.*t419;
t456 = C_d_t.*t121.*t336.*t420;
t457 = C_d_t.*t122.*t337.*t421;
t458 = C_d_t.*t123.*t338.*t422;
t459 = C_d_t.*t135.*t331.*t415;
t460 = C_d_t.*t136.*t332.*t416;
t461 = C_d_t.*t137.*t333.*t417;
t462 = C_d_t.*t138.*t334.*t418;
t463 = C_d_t.*t139.*t335.*t419;
t464 = C_d_t.*t140.*t336.*t420;
t465 = C_d_t.*t141.*t337.*t421;
t466 = C_d_t.*t142.*t338.*t422;
t467 = C_d_t.*t154.*t331.*t415;
t468 = C_d_t.*t155.*t332.*t416;
t469 = C_d_t.*t156.*t333.*t417;
t470 = C_d_t.*t157.*t334.*t418;
t471 = C_d_t.*t158.*t335.*t419;
t472 = C_d_t.*t159.*t336.*t420;
t473 = C_d_t.*t160.*t337.*t421;
t474 = C_d_t.*t161.*t338.*t422;
t354 = t341-1.0;
t355 = t342-1.0;
t356 = t343-1.0;
t357 = t344-1.0;
t358 = t345-1.0;
t359 = t346-1.0;
t360 = t347-1.0;
t361 = t348-1.0;
t362 = t349-1.0;
t424 = E.*t2.*t30.*t116.*t354.*pi.*(5.0./2.0);
xdd_2 = -t292.*(-t424+t451+d_t.*t321.*(Cd_t.*t388.*abs(t388)-Ct_t.*t88.*t203.*t231.*t305.*abs(t88)).*5.0e+2+C_d_t.*t115.*t330.*t363+E.*t2.*t30.*t115.*t353.*pi.*(5.0./2.0));
if nargout > 1
    t425 = E.*t2.*t30.*t117.*t355.*pi.*(5.0./2.0);
    xdd_3 = -t292.*(t424-t425-t451+t452+d_t.*t322.*(Cd_t.*t391.*abs(t391)-Ct_t.*t89.*t204.*t232.*t307.*abs(t89)).*5.0e+2);
end
if nargout > 2
    t426 = E.*t2.*t30.*t118.*t356.*pi.*(5.0./2.0);
    xdd_4 = -t292.*(t425-t426-t452+t453+d_t.*t323.*(Cd_t.*t392.*abs(t392)-Ct_t.*t90.*t205.*t233.*t309.*abs(t90)).*5.0e+2);
end
if nargout > 3
    t427 = E.*t2.*t30.*t119.*t357.*pi.*(5.0./2.0);
    xdd_5 = -t292.*(t426-t427-t453+t454+d_t.*t324.*(Cd_t.*t393.*abs(t393)-Ct_t.*t91.*t206.*t234.*t311.*abs(t91)).*5.0e+2);
end
if nargout > 4
    t428 = E.*t2.*t30.*t120.*t358.*pi.*(5.0./2.0);
    xdd_6 = -t292.*(t427-t428-t454+t455+d_t.*t325.*(Cd_t.*t394.*abs(t394)-Ct_t.*t92.*t207.*t235.*t313.*abs(t92)).*5.0e+2);
end
if nargout > 5
    t429 = E.*t2.*t30.*t121.*t359.*pi.*(5.0./2.0);
    xdd_7 = -t292.*(t428-t429-t455+t456+d_t.*t326.*(Cd_t.*t395.*abs(t395)-Ct_t.*t93.*t208.*t236.*t315.*abs(t93)).*5.0e+2);
end
if nargout > 6
    t430 = E.*t2.*t30.*t122.*t360.*pi.*(5.0./2.0);
    xdd_8 = -t292.*(t429-t430-t456+t457+d_t.*t327.*(Cd_t.*t396.*abs(t396)-Ct_t.*t94.*t209.*t237.*t317.*abs(t94)).*5.0e+2);
end
if nargout > 7
    t431 = E.*t2.*t30.*t123.*t361.*pi.*(5.0./2.0);
    xdd_9 = -t292.*(t430-t431-t457+t458+d_t.*t328.*(Cd_t.*t397.*abs(t397)-Ct_t.*t95.*t210.*t238.*t319.*abs(t95)).*5.0e+2);
end
if nargout > 8
    t432 = E.*t2.*t30.*t124.*t362.*pi.*(5.0./2.0);
    xdd_10 = -t292.*(t431-t432-t458+d_t.*t329.*(Cd_t.*t398.*abs(t398)-Ct_t.*t96.*t124.^2.*t239.*t320.*abs(t96)).*5.0e+2+C_d_t.*t124.*t339.*t423);
end
if nargout > 9
    t433 = E.*t2.*t30.*t135.*t354.*pi.*(5.0./2.0);
    ydd_2 = -t292.*(-t433+t459+d_t.*t321.*(Cd_t.*t389.*abs(t389)-Ct_t.*t97.*t212.*t241.*t305.*abs(t97)).*5.0e+2+C_d_t.*t134.*t330.*t363+E.*t2.*t30.*t134.*t353.*pi.*(5.0./2.0));
end
if nargout > 10
    t434 = E.*t2.*t30.*t136.*t355.*pi.*(5.0./2.0);
    ydd_3 = -t292.*(t433-t434-t459+t460+d_t.*t322.*(Cd_t.*t399.*abs(t399)-Ct_t.*t98.*t213.*t242.*t307.*abs(t98)).*5.0e+2);
end
if nargout > 11
    t435 = E.*t2.*t30.*t137.*t356.*pi.*(5.0./2.0);
    ydd_4 = -t292.*(t434-t435-t460+t461+d_t.*t323.*(Cd_t.*t400.*abs(t400)-Ct_t.*t99.*t214.*t243.*t309.*abs(t99)).*5.0e+2);
end
if nargout > 12
    t436 = E.*t2.*t30.*t138.*t357.*pi.*(5.0./2.0);
    ydd_5 = -t292.*(t435-t436-t461+t462+d_t.*t324.*(Cd_t.*t401.*abs(t401)-Ct_t.*t100.*t215.*t244.*t311.*abs(t100)).*5.0e+2);
end
if nargout > 13
    t437 = E.*t2.*t30.*t139.*t358.*pi.*(5.0./2.0);
    ydd_6 = -t292.*(t436-t437-t462+t463+d_t.*t325.*(Cd_t.*t402.*abs(t402)-Ct_t.*t101.*t216.*t245.*t313.*abs(t101)).*5.0e+2);
end
if nargout > 14
    t438 = E.*t2.*t30.*t140.*t359.*pi.*(5.0./2.0);
    ydd_7 = -t292.*(t437-t438-t463+t464+d_t.*t326.*(Cd_t.*t403.*abs(t403)-Ct_t.*t102.*t217.*t246.*t315.*abs(t102)).*5.0e+2);
end
if nargout > 15
    t439 = E.*t2.*t30.*t141.*t360.*pi.*(5.0./2.0);
    ydd_8 = -t292.*(t438-t439-t464+t465+d_t.*t327.*(Cd_t.*t404.*abs(t404)-Ct_t.*t103.*t218.*t247.*t317.*abs(t103)).*5.0e+2);
end
if nargout > 16
    t440 = E.*t2.*t30.*t142.*t361.*pi.*(5.0./2.0);
    ydd_9 = -t292.*(t439-t440-t465+t466+d_t.*t328.*(Cd_t.*t405.*abs(t405)-Ct_t.*t104.*t219.*t248.*t319.*abs(t104)).*5.0e+2);
end
if nargout > 17
    t441 = E.*t2.*t30.*t143.*t362.*pi.*(5.0./2.0);
    ydd_10 = -t292.*(t440-t441-t466+d_t.*t329.*(Cd_t.*t406.*abs(t406)-Ct_t.*t105.*t143.^2.*t249.*t320.*abs(t105)).*5.0e+2+C_d_t.*t143.*t339.*t423);
end
if nargout > 18
    t442 = E.*t2.*t30.*t154.*t354.*pi.*(5.0./2.0);
    zdd_2 = -t292.*(-t442+t467+d_t.*t321.*(Cd_t.*t390.*abs(t390)-Ct_t.*t106.*t221.*t251.*t305.*abs(t106)).*5.0e+2+C_d_t.*t153.*t330.*t363+E.*t2.*t30.*t153.*t353.*pi.*(5.0./2.0));
end
if nargout > 19
    t443 = E.*t2.*t30.*t155.*t355.*pi.*(5.0./2.0);
    zdd_3 = -t292.*(t442-t443-t467+t468+d_t.*t322.*(Cd_t.*t407.*abs(t407)-Ct_t.*t107.*t222.*t252.*t307.*abs(t107)).*5.0e+2);
end
if nargout > 20
    t444 = E.*t2.*t30.*t156.*t356.*pi.*(5.0./2.0);
    zdd_4 = -t292.*(t443-t444-t468+t469+d_t.*t323.*(Cd_t.*t408.*abs(t408)-Ct_t.*t108.*t223.*t253.*t309.*abs(t108)).*5.0e+2);
end
if nargout > 21
    t445 = E.*t2.*t30.*t157.*t357.*pi.*(5.0./2.0);
    zdd_5 = -t292.*(t444-t445-t469+t470+d_t.*t324.*(Cd_t.*t409.*abs(t409)-Ct_t.*t109.*t224.*t254.*t311.*abs(t109)).*5.0e+2);
end
if nargout > 22
    t446 = E.*t2.*t30.*t158.*t358.*pi.*(5.0./2.0);
    zdd_6 = -t292.*(t445-t446-t470+t471+d_t.*t325.*(Cd_t.*t410.*abs(t410)-Ct_t.*t110.*t225.*t255.*t313.*abs(t110)).*5.0e+2);
end
if nargout > 23
    t447 = E.*t2.*t30.*t159.*t359.*pi.*(5.0./2.0);
    zdd_7 = -t292.*(t446-t447-t471+t472+d_t.*t326.*(Cd_t.*t411.*abs(t411)-Ct_t.*t111.*t226.*t256.*t315.*abs(t111)).*5.0e+2);
end
if nargout > 24
    t448 = E.*t2.*t30.*t160.*t360.*pi.*(5.0./2.0);
    zdd_8 = -t292.*(t447-t448-t472+t473+d_t.*t327.*(Cd_t.*t412.*abs(t412)-Ct_t.*t112.*t227.*t257.*t317.*abs(t112)).*5.0e+2);
end
if nargout > 25
    t449 = E.*t2.*t30.*t161.*t361.*pi.*(5.0./2.0);
    zdd_9 = -t292.*(t448-t449-t473+t474+d_t.*t328.*(Cd_t.*t413.*abs(t413)-Ct_t.*t113.*t228.*t258.*t319.*abs(t113)).*5.0e+2);
end
if nargout > 26
    t450 = E.*t2.*t30.*t162.*t362.*pi.*(5.0./2.0);
    zdd_10 = -t292.*(t449-t450-t474+d_t.*t329.*(Cd_t.*t414.*abs(t414)-Ct_t.*t114.*t162.^2.*t259.*t320.*abs(t114)).*5.0e+2+C_d_t.*t162.*t339.*t423);
end
if nargout > 27
    Tix = [t432;t441;t450];
end
%end

== matlab function External_Forces/Tether/Subsystem1/tether/World to body 1 ==
  data: F_tet_w input; F_tet_b output; phi input; theta input; psi input
function F_tet_b = fcn(F_tet_w,phi,theta,psi)

J_Tinv=[                              cos(psi)*cos(theta)                              cos(theta)*sin(psi)         -sin(theta) 0         0                  0;
 cos(psi)*sin(phi)*sin(theta) - cos(phi)*sin(psi) cos(phi)*cos(psi) + sin(phi)*sin(psi)*sin(theta) cos(theta)*sin(phi) 0         0                  0;
 sin(phi)*sin(psi) + cos(phi)*cos(psi)*sin(theta) cos(phi)*sin(psi)*sin(theta) - cos(psi)*sin(phi) cos(phi)*cos(theta) 0         0                   0;
                                                0                                                0                   0 1         0         -sin(theta);
                                                0                                                0                   0 0  cos(phi) cos(theta)*sin(phi);
                                                0                                                0                   0 0 -sin(phi) cos(phi)*cos(theta)];


F_tet=J_Tinv*[F_tet_w(1) F_tet_w(2) F_tet_w(3) 0 0 0]';
F_tet_b=[F_tet(1) F_tet(2) F_tet(3)]';

== matlab function External_Forces/Ocean currents/World to body  ==
  data: V_current input; V_water output Bus: V_water; eta input
function V_water  = fcn(V_current,eta)

phi = eta.phi; theta = eta.theta; psi = eta.psi;

J_Tinv=[cos(psi)*cos(theta)                                 cos(theta)*sin(psi)                                 -sin(theta);
        cos(psi)*sin(phi)*sin(theta) - cos(phi)*sin(psi)    cos(phi)*cos(psi) + sin(phi)*sin(psi)*sin(theta)    cos(theta)*sin(phi);
        sin(phi)*sin(psi) + cos(phi)*cos(psi)*sin(theta)    cos(phi)*sin(psi)*sin(theta) - cos(psi)*sin(phi)    cos(phi)*cos(theta)];


V_water_b=J_Tinv*[V_current(1) V_current(2) V_current(3)]';
V_water.u = V_water_b(1);
V_water.v = V_water_b(2);
V_water.w = V_water_b(3);

== matlab function External_Forces/Ocean currents/World to body 1 ==
  data: V_water output Bus: V_water
function V_water  = fcn()
V_water.u = 0;
V_water.v = 0;
V_water.w = 0;
